simulink model "Tracking_loop"  (R2025b)
settings: Solver=VariableStepAuto  StartTime=0.0  StopTime=10.0  RelTol=1e-3
settings Model: Creator=samue  LastModifiedBy=samue

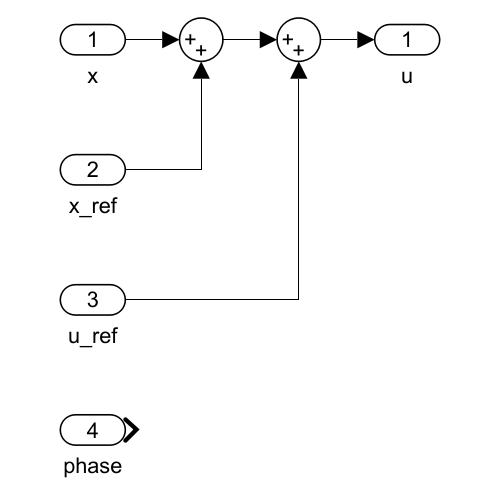
[thumbnail: Simulink's stored preview of the top-level diagram]
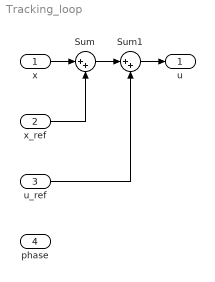
== system Tracking_loop ==
  x : Inport
  x_ref : Inport  Port=2
  u_ref : Inport  Port=3
  phase : Inport  Port=4
  Sum : Sum  Inputs=|++
  Sum1 : Sum  Inputs=|++
  u : Outport
  wires:
  x/1 -> Sum/1
  x_ref/1 -> Sum/2
  Sum1/1 -> u/1
  Sum/1 -> Sum1/1
  u_ref/1 -> Sum1/2
